simulink model "power_hvdc"  (R2013a)
settings: Solver=FixedStepDiscrete  SolverMode=SingleTasking  StartTime=0.0  StopTime=0.8  RelTol=1e-4
undefined symbols (not defined in the file): D1, Delta
libraries: powerlib x28, powerlib_extras x7
Description:
  | Copyright 2008-2013 The MathWorks, Inc.
settings Model: ExtModeTrigMode=oneshot  ExtModeArmWhenConnect=off  ExtModeAutoUpdateStatusClock=off  Creator=MathWorks  LastModifiedBy=nau03113
settings DataIOCC: LimitDataPoints=off  SaveFormat=StructureWithTime  SignalLoggingSaveFormat=ModelDataLogs  SaveOutput=off  TimeSaveName=t  SignalLoggingName=sigsOut
settings OptimizationCC: BlockReduction=off  BooleanDataType=off  ExpressionDepthLimit=2147483647  InitFltsAndDblsToZero=on  EfficientMapNaN2IntZero=off
settings DebuggingCC: CheckExecutionContextPreStartOutputMsg=on  CheckExecutionContextRuntimeOutputMsg=on  SignalResolutionControl=TryResolveAllWithWarning  SolverPrmCheckMsg=none  MultiTaskDSMMsg=warning  MultiTaskCondExecSysMsg=none  FcnCallInpInsideContextMsg=UseLocalSettings
settings HardwareCC: TargetUnknown=on
settings RTWCC: IncludeERTFirstTime=on
settings GRTTargetCC: CombineOutputUpdateFcns=off  GRTInterface=on

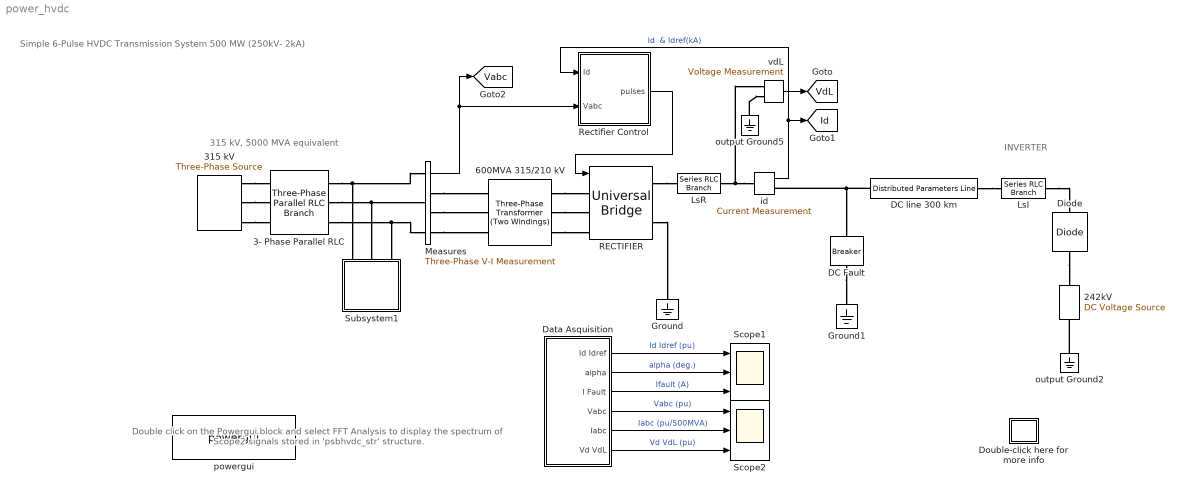
== system power_hvdc ==
  note: INVERTER
  note: Simple 6-Pulse HVDC Transmission System
      | 500 MW (250kV- 2kA)
  note: 315 kV, 5000 MVA equivalent
  note: Double click on the Powergui block
      | and select  FFT Analysis to display
      | the spectrum of Scope2  signals
      | stored in 'psbhvdc_str' structure.
  242kV : powerlib/Electrical Sources/DC Voltage Source  Description=source block  Amplitude=242000  Measurements=None
      settings: AttributesFormatString=\n
  3- Phase Parallel RLC : powerlib/Elements/Three-Phase Parallel RLC Branch  LConnTagsString=A|B|C  RConnTagsString=A|B|C  BranchType=RL  Resistance=12.41  Inductance=23.264e-3  Capacitance=1.0  Measurements=None
  315 kV : powerlib/Electrical Sources/Three-Phase Source  Voltage=315e3  PhaseAngle=0  Frequency=60  InternalConnection=Yg  SpecifyImpedance=off  Resistance=0  Inductance=46.671e-3  ShortCircuitLevel=0  BaseVoltage=0  XRratio=0  BusType=swing  Pref=0  Qref=0  Qmin=-inf  Qmax=inf
  600MVA 315/210 kV : powerlib/Elements/Three-Phase Transformer (Two Windings)  Winding1Connection=Yg  UNITS=pu  NominalPower=[ 600e6 60 ]  Winding1="[ 315e3*0.97 0.0015  0.0 ]"  Winding2Connection=Delta (D1)  Winding2=[ 210e3 0.0015 0.12]  SetSaturation=off  Rm=500  Lm=500  Saturation="[ 0,0  ;  0.005,1.2  ;  1.0,1.4 ]"  Hysteresis=off  DataFile='hysteresis'  SetInitialFlux=off  InitialFluxes=[ 0.8 , -0.8 , 0.7 ]  Measurements=None  MoreParameters=off  BreakLoop=off  DataType=off  TransfoNumber=0
  DC Fault : powerlib/Elements/Breaker  BreakerResistance=0.1  InitialState=0  SnubberResistance=inf  SnubberCapacitance=0  SwitchingTimes=[ 0.5 0.51 ]  External=off  Measurements=Branch current  MoreParameters=off  NoBreakLoop=off
      settings: AttributesFormatString=\n
  DC line 300 km : powerlib/Elements/Distributed Parameters Line  Phases=1  Frequency=60  Resistance=0.015  Inductance=0.792e-3  Capacitance=14.4e-9  Length=300  x1=[-0.00104166666666667 96799.9999940249;-0.000998263888888889 96799.9999940249;-0.000954861111111111 96799.9999940249;-0.000911458333333333 96799.9999940249;-0.000868055555555556 96799.9999940249;-0.000824652777777778 96799.9999940249;-0.00078125 96799.9999940249;-0.000737847222222222 96799.9999940249;-0.000694444444444444 96799.9999940249;-0.000651041666666667 96799.9999940249;-0.000607638888888889 96799.9999940249;-0.000564236111111111 96799.9999940249;-0.000520833333333333 96799.9999940249;-0.000477430555555556 96799.9999940249;-0.000434027777777778 96799.9999940249;-0.000390625 96799.9999940249;-0.000347222222222222 96799.9999940249;-0.000303819444444444 96799.9999940249;-0.000260416666666667 96799.9999940249;-0.000217013888888889 96799.9999940249;-0.000173611111111111 96799.9999940249;-0.000130208333333333 96799.9999940249;-8.68055555555556e-05 96799.9999940249;-4.34027777777778e-05 96799.9999940249]  x2=[-0.00104166666666667 96799.9999940249;-0.000998263888888889 96799.9999940249;-0.000954861111111111 96799.9999940249;-0.000911458333333333 96799.9999940249;-0.000868055555555556 96799.9999940249;-0.000824652777777778 96799.9999940249;-0.00078125 96799.9999940249;-0.000737847222222222 96799.9999940249;-0.000694444444444444 96799.9999940249;-0.000651041666666667 96799.9999940249;-0.000607638888888889 96799.9999940249;-0.000564236111111111 96799.9999940249;-0.000520833333333333 96799.9999940249;-0.000477430555555556 96799.9999940249;-0.000434027777777778 96799.9999940249;-0.000390625 96799.9999940249;-0.000347222222222222 96799.9999940249;-0.000303819444444444 96799.9999940249;-0.000260416666666667 96799.9999940249;-0.000217013888888889 96799.9999940249;-0.000173611111111111 96799.9999940249;-0.000130208333333333 96799.9999940249;-8.68055555555556e-05 96799.9999940249;-4.34027777777778e-05 96799.9999940249]  x3=[-0.00104166666666667 406.863760317022;-0.000998263888888889 406.863760317022;-0.000954861111111111 406.863760317022;-0.000911458333333333 406.863760317022;-0.000868055555555556 406.863760317022;-0.000824652777777778 406.863760317022;-0.00078125 406.863760317022;-0.000737847222222222 406.863760317022;-0.000694444444444444 406.863760317022;-0.000651041666666667 406.863760317022;-0.000607638888888889 406.863760317022;-0.000564236111111111 406.863760317022;-0.000520833333333333 406.863760317022;-0.000477430555555556 406.863760317022;-0.000434027777777778 406.863760317022;-0.000390625 406.863760317022;-0.000347222222222222 406.863760317022;-0.000303819444444444 406.863760317022;-0.000260416666666667 406.863760317022;-0.000217013888888889 406.863760317022;-0.000173611111111111 406.863760317022;-0.000130208333333333 406.863760317022;-8.68055555555556e-05 406.863760317022;-4.34027777777778e-05 406.863760317022]  x4=[-0.00104166666666667 406.863760317022;-0.000998263888888889 406.863760317022;-0.000954861111111111 406.863760317022;-0.000911458333333333 406.863760317022;-0.000868055555555556 406.863760317022;-0.000824652777777778 406.863760317022;-0.00078125 406.863760317022;-0.000737847222222222 406.863760317022;-0.000694444444444444 406.863760317022;-0.000651041666666667 406.863760317022;-0.000607638888888889 406.863760317022;-0.000564236111111111 406.863760317022;-0.000520833333333333 406.863760317022;-0.000477430555555556 406.863760317022;-0.000434027777777778 406.863760317022;-0.000390625 406.863760317022;-0.000347222222222222 406.863760317022;-0.000303819444444444 406.863760317022;-0.000260416666666667 406.863760317022;-0.000217013888888889 406.863760317022;-0.000173611111111111 406.863760317022;-0.000130208333333333 406.863760317022;-8.68055555555556e-05 406.863760317022;-4.34027777777778e-05 406.863760317022]  x5=0.00101312980412186  Measurements=None
      settings: AttributesFormatString=\n
  Data Asquisition : Subsystem
  Diode : powerlib/Power Electronics/Diode  Ron=0.01  Lon=0  Vf=0.8  IC=0  UseSnubber=off  Rs=1000  Cs=0.05e-6  Measurements=off
  Double-click here for more info : Subsystem
      settings: OpenFcn=showdemo(bdroot(gcb))
      mask Display: disp('?')
  Ground : powerlib/Elements/Ground  LConnTagsString=a
  Ground1 : powerlib/Elements/Ground  LConnTagsString=a
  LsI : powerlib/Elements/Series RLC Branch  LConnTagsString=__new0  RConnTagsString=__new0  BranchType=RL  Resistance=.5  Inductance=.5  SetiL0=off  InitialCurrent=0  Capacitance=1.0  Setx0=off  InitialVoltage=0  Measurements=None
  "LsR " : powerlib/Elements/Series RLC Branch  LConnTagsString=__new0  RConnTagsString=__new0  BranchType=RL  Resistance=.5  Inductance=.5  SetiL0=off  InitialCurrent=0  Capacitance=1.0  Setx0=off  InitialVoltage=0  Measurements=None
  Measures : powerlib/Measurements/Three-Phase V-I Measurement  VoltageMeasurement=phase-to-ground  SetLabelV=off  LabelV=V1  Vpu=on  VpuLL=off  CurrentMeasurement=yes  SetLabelI=on  LabelI=Iabc  Ipu=on  Pbase=500e6  Vbase=315e3  OutputType=Magnitude  PhasorSimulation=off  PSBequivalent=0
  RECTIFIER : powerlib/Power Electronics/Universal Bridge  Arms=3  SnubberResistance=2000  SnubberCapacitance=50e-9  Device=Thyristors  Ron=1e-3  Lon=0  ForwardVoltages="[  0.8  0.8  ]"  ForwardVoltage=0  GTOparameters=[ 10e-6 , 20e-6 ]  IGBTparameters=[ 1e-6 , 2e-6 ]  Measurements=UAB UBC UCA UDC voltages  Measurements_2=None  converterType=Rectifier
  Rectifier Control : Subsystem
  Scope1 : Scope  NumInputPorts=3
      settings: TimeRange=0.8  YMin=-0.25~0~-500  YMax=2~170~6000
  Scope2 : Scope  NumInputPorts=3
      settings: TimeRange=0.8  YMin=-1.5~-3~-1.5  YMax=1.5~3~2  SaveName=psbhvdc_str
  Subsystem1 : Subsystem
      mask Display: disp('AC filters \n(320 Mvar)')
  id : powerlib/Measurements/Current Measurement  Tag=PoWeRsYsTeMmEaSuReMeNt  PhasorSimulation=off  OutputType=Complex  PSBequivalent=0
  output Ground2 : powerlib/Elements/Ground  LConnTagsString=a
  output Ground5 : powerlib/Elements/Ground  LConnTagsString=a
  powergui : powerlib/powergui  Priority=2  SimulationMode=Discrete  SolverType=Tustin  SampleTime=1/360/64  frequency=60  SPID=off  DisableSnubberDevices=off  DisableRonSwitches=off  DisableVfSwitches=off  SwTol=0  Interpol=off  DisplayEquations=off  frequencyindice=60  Pbase=100e6  ErrMax=1e-4  Iterations=50  UnitsV=kV  UnitsW=MW  FunctionMessages=off  echomessages=off  HookPort=off  EnableUseOfTLC=off  x0status=blocks  RestoreLinks=warning  ResistiveCurrentMeasurement=off  Frange=[0:2:500]  Ylog=off  Xlog=off  ShowGrid=off  save=off  variable=ZData  structure=psbhvdc_str  ZoomFFT=on  StartTime=0.2  cycles=2  DisplayStyle=2  fundamental=60  FreqAxis=on  MaxFrequency=4000  frequencyindicesteady=1  RmsSteady=1  display=off  Ts=0  methode=off
  vdL : powerlib/Measurements/Voltage Measurement  Tag=PoWeRsYsTeMmEaSuReMeNt  PhasorSimulation=off  OutputType=Complex  PSBequivalent=0
  tag scope: Id=global, Vabc=global, VdL=global
  wires:
  Data Asquisition/6(Vd VdL) -> Scope2/3  "Vd VdL (pu)"
  Data Asquisition/1("Id Idref ") -> Scope1/1  "Id Idref (pu)"
  Data Asquisition/3(I Fault) -> Scope1/3  "Ifault (A)"
  Data Asquisition/2(alpha) -> Scope1/2  "alpha (deg.)"
  Data Asquisition/4(Vabc) -> Scope2/1  "Vabc (pu)"
  Data Asquisition/5(Iabc) -> Scope2/2  "Iabc (pu/500MVA)"
  Rectifier Control/1(pulses) -> RECTIFIER/1
  id/1 -> Rectifier Control/1(Id), [Id]  "Id  & Idref(kA)"
  Measures/1 -> [Vabc], Rectifier Control/2(Vabc)
  vdL/1 -> [VdL]
  connections:
  RECTIFIER/RConn1 -- "LsR "/LConn1
  RECTIFIER/RConn2 -- Ground/LConn1
  600MVA 315/210 kV/RConn1 -- RECTIFIER/LConn1
  600MVA 315/210 kV/RConn2 -- RECTIFIER/LConn2
  600MVA 315/210 kV/RConn3 -- RECTIFIER/LConn3
  Measures/RConn1 -- 600MVA 315/210 kV/LConn1
  Measures/RConn2 -- 600MVA 315/210 kV/LConn2
  Measures/RConn3 -- 600MVA 315/210 kV/LConn3
  DC line 300 km/RConn1 -- LsI/LConn1
  DC line 300 km/LConn1 -- id/RConn1 -- DC Fault/LConn1
  "LsR "/RConn1 -- id/LConn1 -- vdL/LConn1
  output Ground5/LConn1 -- vdL/LConn2
  DC Fault/RConn1 -- Ground1/LConn1
  output Ground2/LConn1 -- 242kV/LConn1
  LsI/RConn1 -- Diode/LConn1
  315 kV/RConn1 -- 3- Phase Parallel RLC/LConn1
  315 kV/RConn2 -- 3- Phase Parallel RLC/LConn2
  315 kV/RConn3 -- 3- Phase Parallel RLC/LConn3
  Diode/RConn1 -- 242kV/RConn1
  3- Phase Parallel RLC/RConn2 -- Measures/LConn2 -- Subsystem1/LConn2
  3- Phase Parallel RLC/RConn1 -- Measures/LConn1 -- Subsystem1/LConn1
  3- Phase Parallel RLC/RConn3 -- Measures/LConn3 -- Subsystem1/LConn3

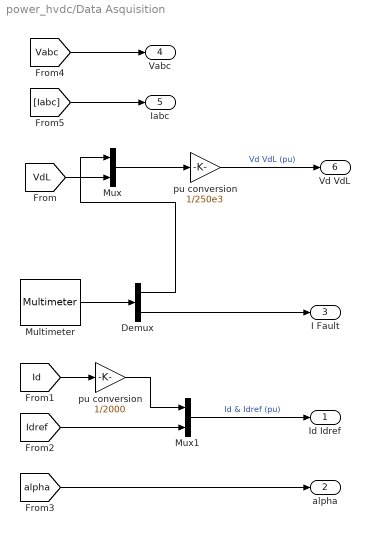
== system power_hvdc/Data Asquisition ==
  Demux : Demux  Outputs=2
  Multimeter : powerlib/Measurements/Multimeter  Tag=PoWeRsYsTeMmEaSuReMeNt  PhasorSimulation=off  OutputType=Magnitude  sel=[4 5]  L=5  Gain=[1 1]  yselected={'Udc: RECTIFIER','Ib: DC Fault'};  PSBOutputType=1  PSBequivalent=0  AxesSetting=[0,0.1,-100,100]  Display=0  SavedBlockNames={}
      settings: AttributesFormatString=\n
  Mux : Mux  Inputs=2
  Mux1 : Mux  Inputs=2
  pu conversion : Gain  Gain=1/2000  SaturateOnIntegerOverflow=on  OutDataTypeStr=Inherit: Same as input  ParamDataTypeStr=Inherit: Same as input
  "pu conversion " : Gain  Gain=1/250e3  SaturateOnIntegerOverflow=on  OutDataTypeStr=Inherit: Same as input  ParamDataTypeStr=Inherit: Same as input
  "Id Idref " : Outport
  alpha : Outport  Port=2
  I Fault : Outport  Port=3
  Vabc : Outport  Port=4
  Iabc : Outport  Port=5
  Vd VdL : Outport  Port=6
  wires:
  Mux/1 -> "pu conversion "/1
  [VdL] -> Mux/2
  [Id] -> pu conversion/1
  Mux1/1 -> "Id Idref "/1  "Id & Idref (pu)"
  [Idref] -> Mux1/2
  Demux/2 -> I Fault/1
  Demux/1 -> Mux/1
  [alpha] -> alpha/1
  [Vabc] -> Vabc/1
  [Iabc] -> Iabc/1
  "pu conversion "/1 -> Vd VdL/1  "Vd VdL (pu)"
  pu conversion/1 -> Mux1/1
  Multimeter/1 -> Demux/1

== system power_hvdc/Double-click here for more info ==

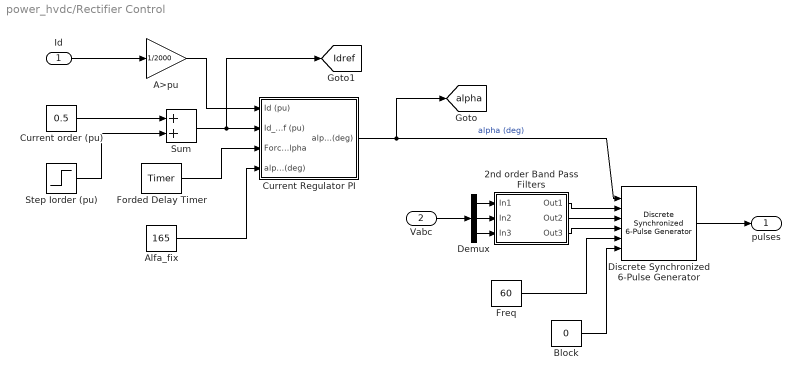
== system power_hvdc/Rectifier Control ==
  Id : Inport
  Vabc : Inport  Port=2
  2nd order Band Pass Filters : Subsystem
      mask Display: disp(' Fo=60 Hz\n\nBW=30 Hz')
  A>pu : Gain  Gain=1/2000  SaturateOnIntegerOverflow=on  OutDataTypeStr=Inherit: Same as input  ParamDataTypeStr=Inherit: Same as input
  Alfa_fix : Constant  Value=165
  Block : Constant  Value=0
  Current Regulator PI : Subsystem
  Current order (pu) : Constant  Value=0.5
  Demux : Demux  Outputs=3
  Discrete Synchronized 6-Pulse Generator : powerlib_extras/Discrete  Control Blocks/Discrete Synchronized 6-Pulse Generator  pwidth=70  Double_Pulse=off  Ts=1/360/64
  Forded Delay Timer : powerlib_extras/Control  Blocks/Timer  t=[ 0.55 0.57]  e="[1 0  ]"
  Freq : Constant  Value=60
  "Step Iorder (pu)  " : Step  Time=0.3  After=0.6  SampleTime=0  ZeroCross=off
  Sum : Sum  SaturateOnIntegerOverflow=on  InputSameDT=on  OutDataTypeStr=Inherit: Same as first input
  pulses : Outport
  tag scope: Idref=global, alpha=global
  wires:
  Demux/1 -> 2nd order Band Pass Filters/1(In1)
  Demux/3 -> 2nd order Band Pass Filters/3(In3)
  Demux/2 -> 2nd order Band Pass Filters/2(In2)
  2nd order Band Pass Filters/2(Out2) -> Discrete Synchronized 6-Pulse Generator/3
  2nd order Band Pass Filters/1(Out1) -> Discrete Synchronized 6-Pulse Generator/2
  2nd order Band Pass Filters/3(Out3) -> Discrete Synchronized 6-Pulse Generator/4
  Block/1 -> Discrete Synchronized 6-Pulse Generator/6
  Freq/1 -> Discrete Synchronized 6-Pulse Generator/5
  Vabc/1 -> Demux/1
  Discrete Synchronized 6-Pulse Generator/1 -> pulses/1
  Current order (pu)/1 -> Sum/1
  "Step Iorder (pu)  "/1 -> Sum/2
  Sum/1 -> Current Regulator PI/2(Id_ref (pu)), [Idref]
  A>pu/1 -> Current Regulator PI/1(Id (pu))
  Current Regulator PI/1(alpha (deg)) -> Discrete Synchronized 6-Pulse Generator/1, [alpha]  "alpha (deg)"
  Alfa_fix/1 -> Current Regulator PI/4(alpha_fix(deg))
  Forded Delay Timer/1 -> Current Regulator PI/3(Forced_alpha)
  Id/1 -> A>pu/1

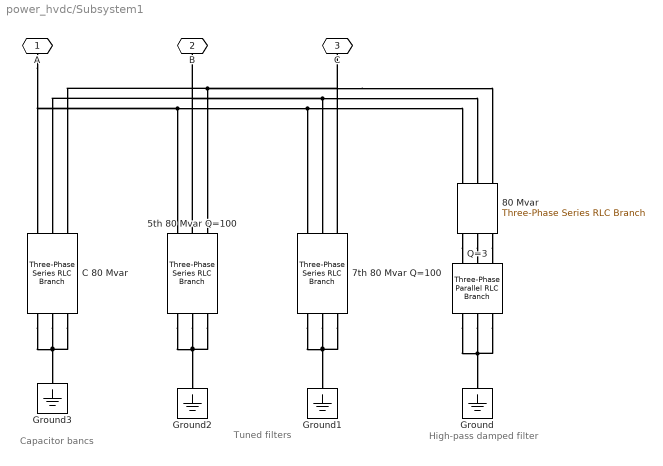
== system power_hvdc/Subsystem1 ==
  note: High-pass
      | damped filter
  note: Tuned filters
  note: Capacitor bancs
  "5th 80 Mvar Q=100 " : powerlib/Elements/Three-Phase Series RLC Branch  LConnTagsString=A|B|C  RConnTagsString=A|B|C  BranchType=RLC  Resistance=2.48  Inductance=131.5e-3  Capacitance=2.14e-6  Measurements=None
  7th 80 Mvar Q=100 : powerlib/Elements/Three-Phase Series RLC Branch  LConnTagsString=A|B|C  RConnTagsString=A|B|C  BranchType=RLC  Resistance=1.77  Inductance=67.1e-3  Capacitance=2.14e-6  Measurements=None
  80 Mvar : powerlib/Elements/Three-Phase Series RLC Branch  LConnTagsString=A|B|C  RConnTagsString=A|B|C  BranchType=C  Resistance=1.0  Inductance=1.0  Capacitance=2.14e-6  Measurements=None
  C 80 Mvar : powerlib/Elements/Three-Phase Series RLC Branch  LConnTagsString=A|B|C  RConnTagsString=A|B|C  BranchType=C  Resistance=1.0  Inductance=1.0  Capacitance=2.14e-6  Measurements=None
  Ground{,1..3} (4 alike) : powerlib/Elements/Ground  LConnTagsString=a
  Q=3 : powerlib/Elements/Three-Phase Parallel RLC Branch  LConnTagsString=A|B|C  RConnTagsString=A|B|C  BranchType=RL  Resistance=225.6  Inductance=27.2e-3  Capacitance=1.0  Measurements=None
  A : PMIOPort  Port=1  Side=Left
  B : PMIOPort  Port=2  Side=Left
  C : PMIOPort  Port=3  Side=Left
  connections:
  80 Mvar/RConn3 -- Q=3/LConn3
  80 Mvar/RConn2 -- Q=3/LConn2
  80 Mvar/RConn1 -- Q=3/LConn1
  "5th 80 Mvar Q=100 "/RConn3 -- "5th 80 Mvar Q=100 "/RConn2 -- Ground2/LConn1 -- "5th 80 Mvar Q=100 "/RConn1
  C 80 Mvar/RConn3 -- C 80 Mvar/RConn2 -- Ground3/LConn1 -- C 80 Mvar/RConn1
  Q=3/RConn2 -- Ground/LConn1 -- Q=3/RConn3 -- Q=3/RConn1
  7th 80 Mvar Q=100/RConn3 -- 7th 80 Mvar Q=100/RConn2 -- Ground1/LConn1 -- 7th 80 Mvar Q=100/RConn1
  A/RConn1 -- C 80 Mvar/LConn1 -- 80 Mvar/LConn1 -- 7th 80 Mvar Q=100/LConn1 -- "5th 80 Mvar Q=100 "/LConn1
  "5th 80 Mvar Q=100 "/LConn2 -- B/RConn1 -- C 80 Mvar/LConn2 -- 80 Mvar/LConn2 -- 7th 80 Mvar Q=100/LConn2
  7th 80 Mvar Q=100/LConn3 -- C/RConn1 -- 80 Mvar/LConn3 -- C 80 Mvar/LConn3 -- "5th 80 Mvar Q=100 "/LConn3

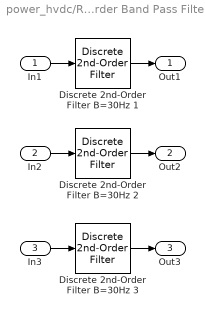
== system power_hvdc/Rectifier Control/2nd order Band Pass Filters ==
  In1 : Inport
  In2 : Inport  Port=2
  In3 : Inport  Port=3
  Discrete 2nd-Order Filter B=30Hz 1 : powerlib_extras/Discrete  Control Blocks/Discrete  2nd-Order Filter  FilterType=Bandpass  Fo=60  Zeta=0.25  Ts=1/360/64  Initialize=on  Vac_Init=[0.8 -25 60]  Vdc_Init=-0.4  PlotResponse=off  param1=[1 500 0.1]
  Discrete 2nd-Order Filter B=30Hz 2 : powerlib_extras/Discrete  Control Blocks/Discrete  2nd-Order Filter  FilterType=Bandpass  Fo=60  Zeta=0.25  Ts=1/360/64  Initialize=on  Vac_Init=[0.8 -25 60]  Vdc_Init=-0.4  PlotResponse=off  param1=[1 500 0.1]
  Discrete 2nd-Order Filter B=30Hz 3 : powerlib_extras/Discrete  Control Blocks/Discrete  2nd-Order Filter  FilterType=Bandpass  Fo=60  Zeta=0.25  Ts=1/360/64  Initialize=on  Vac_Init=[0.8 -25 60]  Vdc_Init=-0.4  PlotResponse=off  param1=[1 500 0.1]
  Out1 : Outport
  Out2 : Outport  Port=2
  Out3 : Outport  Port=3
  wires:
  Discrete 2nd-Order Filter B=30Hz 1/1 -> Out1/1
  In1/1 -> Discrete 2nd-Order Filter B=30Hz 1/1
  In2/1 -> Discrete 2nd-Order Filter B=30Hz 2/1
  In3/1 -> Discrete 2nd-Order Filter B=30Hz 3/1
  Discrete 2nd-Order Filter B=30Hz 2/1 -> Out2/1
  Discrete 2nd-Order Filter B=30Hz 3/1 -> Out3/1

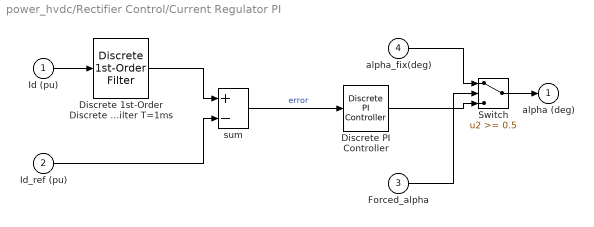
== system power_hvdc/Rectifier Control/Current Regulator PI ==
  Id (pu) : Inport
  Id_ref (pu) : Inport  Port=2
  Forced_alpha : Inport  Port=3
  alpha_fix(deg) : Inport  Port=4
  Discrete 1st-Order Discrete Filter T=1ms : powerlib_extras/Discrete  Control Blocks/Discrete 1st-Order Filter  FilterType=Lowpass  Tc=1e-3  Ts=1/360/64  Initialize=off  Vac_Init=[0.8 -25 60]  Vdc_Init=-0.4  PlotResponse=off  param1=[1 500 0.1]
  Discrete PI Controller : powerlib_extras/Discrete  Control Blocks/Discrete PI Controller  Kp=65  Ki=5000  Par_Limits=[165 5]  Init=90  Ts=1/360/64
  Switch : Switch  Threshold=0.5  ZeroCross=off  InputSameDT=on
  sum : Sum  Inputs=+-  SaturateOnIntegerOverflow=on  InputSameDT=on  OutDataTypeStr=Inherit: Same as first input
  alpha (deg) : Outport  InitialOutput=0
  wires:
  Id_ref (pu)/1 -> sum/2
  Discrete 1st-Order Discrete Filter T=1ms/1 -> sum/1
  Id (pu)/1 -> Discrete 1st-Order Discrete Filter T=1ms/1
  sum/1 -> Discrete PI Controller/1  "error"
  Forced_alpha/1 -> Switch/2
  Switch/1 -> alpha (deg)/1
  alpha_fix(deg)/1 -> Switch/1
  Discrete PI Controller/1 -> Switch/3
